simulink model "experiment_supervisor"  (R2023a)
settings: Solver=FixedStepDiscrete  StartTime=0.0  StopTime=inf  FixedStep=Ts  RelTol=1e-3
model workspace (MAT data in the model file):
  Ts = Simulink.Parameter
  Ts.Value = 0.01
  Ts.DataType = 'auto'
  Ts.DocUnits = 's'
  Ts.Complexity = 'real'
  Ts.Dimensions = [1 1]
  board_ID = Simulink.Parameter
  board_ID.Value = 1
  board_ID.DataType = 'auto'
  board_ID.Complexity = 'real'
  board_ID.Dimensions = [1 1]
undefined symbols (not defined in the file or in its folder): CAN_ANGLE_DEG2ICUB, CAN_VOLT_REF_GAIN, CAN_VOLT_REF_SHIFT, canChannel
libraries: canmsglib x12, canlib x4
settings Model: DataDictionary=EmbeddedBoardDD.sldd  Creator=upattacini  LastModifiedBy=mfussi
settings SolverCC: AlgebraicLoopSolver=TrustRegion  DecoupledContinuousIntegration=on  MinimalZcImpactIntegration=on
settings OptimizationCC: ReuseModelBlockBuffer=off  SimCompilerOptimization=on
settings DebuggingCC: UnconnectedInputMsg=warning  UnconnectedOutputMsg=warning  UnconnectedLineMsg=warning  ArithmeticOperatorsInVariantConditions=warning
settings HardwareCC: ProdBitPerLong=64  ProdHWDeviceType=Intel->x86-64 (Linux 64)
settings ModelReferenceCC: EnableRefExpFcnMdlSchedulingChecks=on
settings SFSimCC: SimUseLocalCustomCode=off  CustomCodeUndefinedFunction=UseInterfaceOnly
settings RTWCC: Description=Simulink Desktop Real-Time  SystemTargetFile=sldrt.tlc  TemplateMakefile=sldrt.tmf  RTWUseLocalCustomCode=off  RTWCompilerOptimization=on  DLArmComputeVersion=19.05
settings CodeAppCC: MaxIdLength=95
settings SimulinkDesktopRealTimeCC: TargetLibSuffix=_sldrt.a  TargetPreCompLibLocation=C:\Program Files\MATLAB\R2023a\toolbox\sldrt\lib\win64

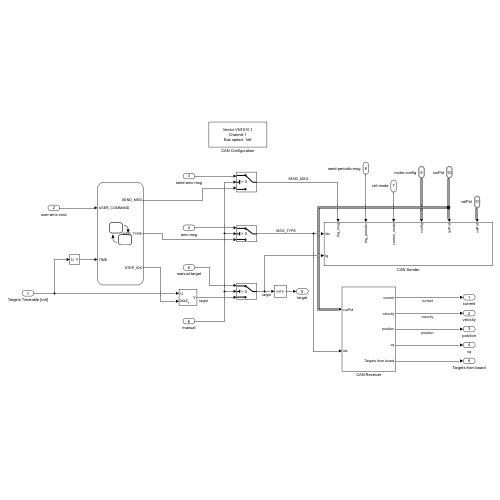
[thumbnail: Simulink's stored preview of the top-level diagram]
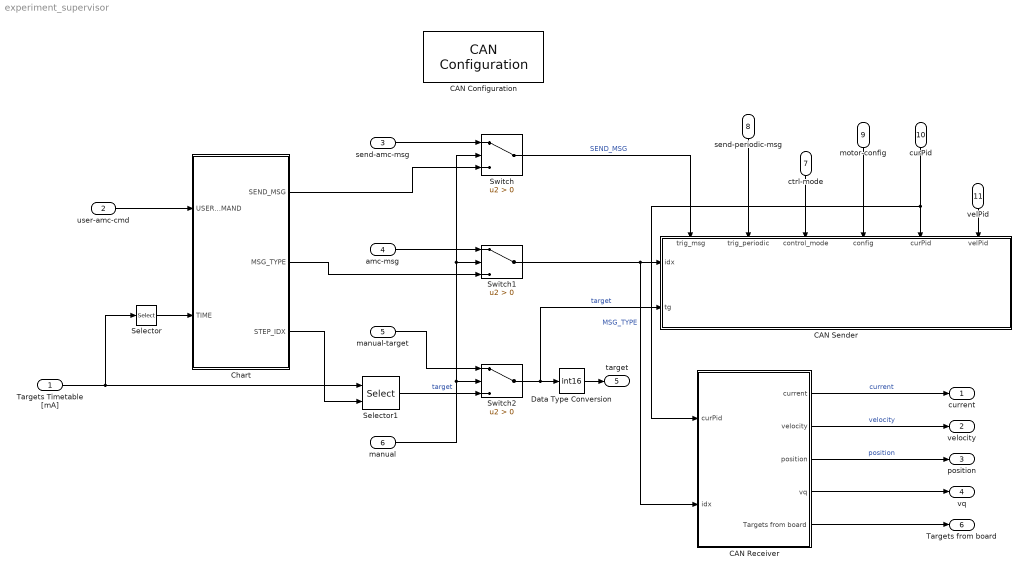
== system experiment_supervisor ==
  Targets Timetable [mA] : Inport  PortDimensions=[2, 8]
  user-amc-cmd : Inport  Port=2
  send-amc-msg : Inport  Port=3
  amc-msg : Inport  Port=4
  manual-target : Inport  Port=5
  manual : Inport  Port=6
  ctrl-mode : Inport  Port=7
  send-periodic-msg : Inport  Port=8
  motor-config : Inport  Port=9  OutDataTypeStr=Bus: MotorConfig
  curPid : Inport  Port=10  OutDataTypeStr=Bus: PIDConfig
  velPid : Inport  Port=11  OutDataTypeStr=Bus: PIDConfig
  CAN Configuration : canlib/CAN Configuration  BlockHandle=1472.0001  Device=Vector VN1610 1 (Channel 1)  DeviceMenu=Vector VN1610 1 (Channel 1)  ObjConstructor=canChannel('Vector', 'VN1610 1', 1)  BusSpeed=1e6  EnableBitParameters=off  SJW=1  TSEG1=4  TSEG2=3  NSamples=1  AckMode=Normal
  CAN Receiver : Subsystem
  CAN Sender : Subsystem
      settings: PortSchema="{\"entries\":[{\"content\":{\"sides\":[{\"content\":{\"connectorIds\":[\"In1\",\"In2\"]},\"type\":\"ConnectorPlacement.EquallySpacedRectSide\",\"uuid\":\"bdd6ce9e-9b65-4aba-9b48-f09f8c1326bb\"},{\"content\":{\"connectorIds\":[],\"side\":\"RIGHT\"},\"type\":\"ConnectorPlacement.EquallySpacedRectSide\",\"uuid\":\"141c9ef5-f742-47fc-b635-015c7474b58f\"},{\"content\":{\"connectorIds\":[\"In3\",\"In4\",\"In5\",\"In6\",\"In7\",\"In8\"],\"side\":\"TOP\"},\"type\":\"ConnectorPlacement.EquallySpacedRectSide\",\"uuid\":\"624889ac-74c5-4b05-9d21-0587daea952f\"}]},\"type\":\"ConnectorPlacement.EquallySpacedConnector\",\"uuid\":\"a748afda-e52d-41b4-a312-ee668058905d\"}],\"packageUris\":[\"http://schema.mathworks.com/mf0/Connector/R2020b\"],\"version\":\"1.0\"}"
  Chart : Stateflow chart  TreatAsAtomicUnit=on
      settings: PortSchema="{\"entries\":[{\"content\":{\"sides\":[{\"content\":{\"connectorIds\":[\"In1\",\"In2\"]},\"type\":\"ConnectorPlacement.EquallySpacedRectSide\",\"uuid\":\"3f3ecf7a-eca8-49e2-a594-4c8df01bcae2\"},{\"content\":{\"connectorIds\":[\"Out2\",\"Out1\",\"Out3\"],\"side\":\"RIGHT\"},\"type\":\"ConnectorPlacement.EquallySpacedRectSide\",\"uuid\":\"2e405059-6050-4daf-b42b-e1c8d6f3a572\"},{\"content\":{\"connectorIds\":[],\"side\":\"TOP\"},\"type\":\"ConnectorPlacement.EquallySpacedRectSide\",\"uuid\":\"8705f6e5-e301-4990-b24d-44270950b42f\"}]},\"type\":\"ConnectorPlacement.EquallySpacedConnector\",\"uuid\":\"46b9b7aa-14e0-48f8-b8fe-455c7835f2bb\"}],\"packageUris\":[\"http://schema.mathworks.com/mf0/Connector/R2020b\"],\"version\":\"1.0\"}"
  Data Type Conversion : DataTypeConversion  OutDataTypeStr=int16  SaturateOnIntegerOverflow=off  RndMeth=Floor
  Selector : Selector  NumberOfDimensions=2  InputPortWidth=2  IndexOptions=Index vector (dialog),Select all  Indices=1,2  OutputSizes=1,6
  Selector1 : Selector  NumberOfDimensions=2  InputPortWidth=2  IndexOptions=Index vector (dialog),Index vector (port)  Indices=2,2  OutputSizes=1,6
  Switch : Switch  Criteria=u2 > Threshold  SaturateOnIntegerOverflow=off  InputSameDT=off
  Switch1 : Switch  Criteria=u2 > Threshold  SaturateOnIntegerOverflow=off  InputSameDT=off
  Switch2 : Switch  Criteria=u2 > Threshold  SaturateOnIntegerOverflow=off  InputSameDT=off
  current : Outport
  velocity : Outport  Port=2
  position : Outport  Port=3
  vq : Outport  Port=4
  target : Outport  Port=5
  Targets from board : Outport  Port=6
  wires:
  Chart/1(MSG_TYPE) -> Switch1/3
  amc-msg/1 -> Switch1/1
  user-amc-cmd/1 -> Chart/1(USER_COMMAND)
  Chart/2(SEND_MSG) -> Switch/3
  send-amc-msg/1 -> Switch/1
  Switch/1 -> CAN Sender/3(trig_msg)  "SEND_MSG"
  Switch1/1 -> CAN Sender/1(idx), CAN Receiver/2(idx)  "MSG_TYPE"
  Chart/3(STEP_IDX) -> Selector1/2
  Selector/1 -> Chart/2(TIME)
  Switch2/1 -> Data Type Conversion/1, CAN Sender/2(tg)  "target"
  manual-target/1 -> Switch2/1
  Selector1/1 -> Switch2/3  "target"
  manual/1 -> Switch/2, Switch1/2, Switch2/2
  Targets Timetable [mA]/1 -> Selector/1, Selector1/1
  CAN Receiver/1(current) -> current/1  "current"
  CAN Receiver/2(velocity) -> velocity/1  "velocity"
  CAN Receiver/3(position) -> position/1  "position"
  CAN Receiver/4(vq) -> vq/1
  ctrl-mode/1 -> CAN Sender/5(control_mode)
  send-periodic-msg/1 -> CAN Sender/4(trig_periodic)
  Data Type Conversion/1 -> target/1
  CAN Receiver/5(Targets from board) -> Targets from board/1
  velPid/1 -> CAN Sender/8(velPid)
  curPid/1 -> CAN Sender/7(curPid), CAN Receiver/1(curPid)
  motor-config/1 -> CAN Sender/6(config)

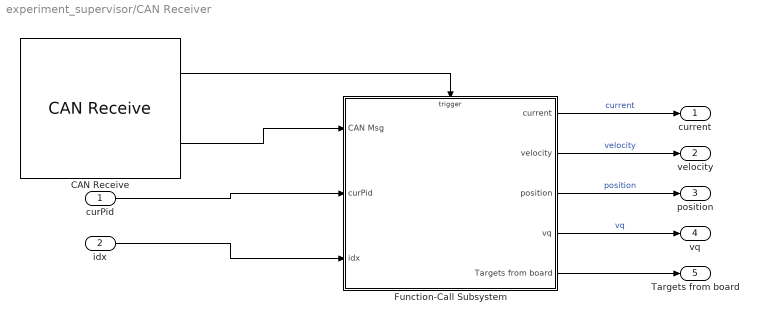
== system experiment_supervisor/CAN Receiver ==
  curPid : Inport  OutDataTypeStr=Bus: PIDConfig
  idx : Inport  Port=2
  CAN Receive : canlib/CAN Receive  BlockHandle=1483.0001  Device=Vector VN1610 1 (Channel 1)  DeviceMenu=Vector VN1610 1 (Channel 1)  ObjConstructor=canChannel('Vector', 'VN1610 1', 1)  EnableStandardIDsFilter=off  StdIDsCombo=Allow all  StandardIDs=0  EnableExtendedIDsFilter=off  ExtIDsCombo=Allow all  ExtendedIDs=0  SampleTime=Ts  MsgsPerTimestep=all  InternalFilterUpdateStatus=on  BusOutput=on
  Function-Call Subsystem : Subsystem  TreatAsAtomicUnit=on
  current : Outport
  velocity : Outport  Port=2
  position : Outport  Port=3
  vq : Outport  Port=4
  Targets from board : Outport  Port=5
  wires:
  CAN Receive/1 -> Function-Call Subsystem/Trigger
  CAN Receive/2 -> Function-Call Subsystem/1(CAN Msg)
  idx/1 -> Function-Call Subsystem/3(idx)
  Function-Call Subsystem/1(current) -> current/1  "current"
  Function-Call Subsystem/2(velocity) -> velocity/1  "velocity"
  Function-Call Subsystem/3(position) -> position/1  "position"
  Function-Call Subsystem/4(vq) -> vq/1  "vq"
  Function-Call Subsystem/5(Targets from board) -> Targets from board/1
  curPid/1 -> Function-Call Subsystem/2(curPid)

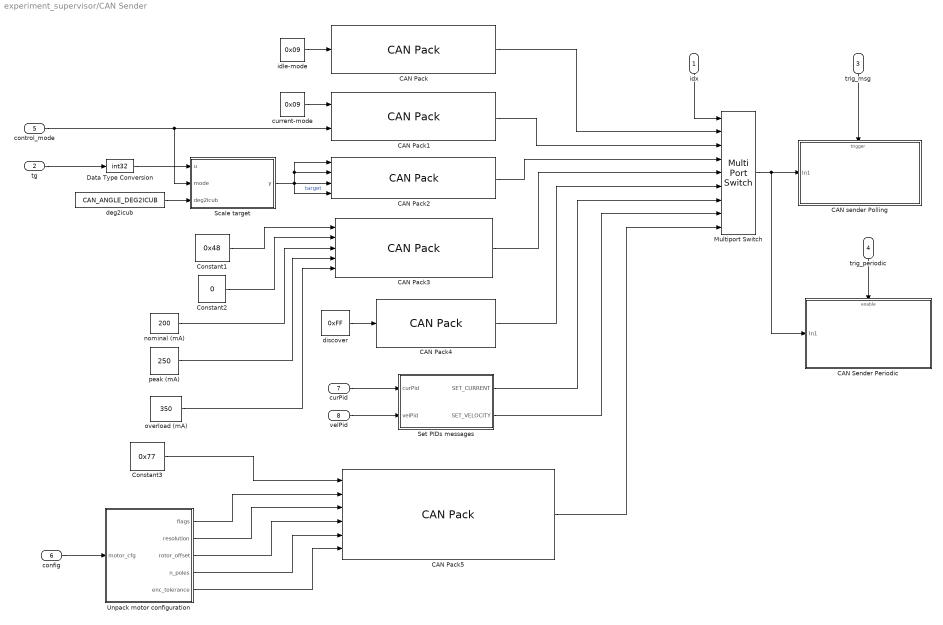
== system experiment_supervisor/CAN Sender ==
  idx : Inport
  tg : Inport  Port=2
  trig_msg : Inport  Port=3
  trig_periodic : Inport  Port=4
  control_mode : Inport  Port=5
  config : Inport  Port=6  OutDataTypeStr=Bus: MotorConfig
  curPid : Inport  Port=7
  velPid : Inport  Port=8
  CAN Pack : canmsglib/CAN Pack  MsgList=(none)  MsgName=CAN Idle  MsgIDType=Standard (11-bit identifier)  MsgIdentifier=board_ID  MsgLength=2  Remote=off  ApplyMinMax=off  BusOutput=on  SignalInfo={ 'Idle', '0', '16', 'LE', 'unsigned', 'Standard', '0', '1', '0', '-Inf', 'Inf' }
      settings: DataFormat=manually specified signals
  CAN Pack1 : canmsglib/CAN Pack  MsgList=(none)  MsgName=SET Control Mode  MsgIDType=Standard (11-bit identifier)  MsgIdentifier=board_ID  MsgLength=2  Remote=off  ApplyMinMax=off  BusOutput=on  SignalInfo={ 'CMD', '0', '8', 'LE', 'unsigned', 'Standard', '0', '1', '0', '-Inf', 'Inf'; 'CTRL', '8', '8', 'LE', 'signed', 'Standard', '0', '1', '0', '-Inf', 'Inf' }
      settings: DataFormat=manually specified signals
  CAN Pack2 : canmsglib/CAN Pack  MsgList=(none)  MsgName=CAN Target  MsgIDType=Standard (11-bit identifier)  MsgIdentifier=0x10F  MsgLength=8  Remote=off  ApplyMinMax=off  BusOutput=on  SignalInfo={ 'Target 1', '0', '16', 'LE', 'signed', 'Standard', '0', '1', '0', '-Inf', 'Inf'; 'Target 2', '16', '16', 'LE', 'signed', 'Standard', '0', '1', '0', '-Inf', 'Inf'; 'Target 3', '32', '16', 'LE', 'signed', 'Standard', '0', '1', '0', '-Inf', 'Inf'; 'Target 4', '48', '16', 'LE', 'signed', 'Standard', '0', '1', '0', '-Inf', 'Inf' }
      settings: DataFormat=manually specified signals
  CAN Pack3 : canmsglib/CAN Pack  MsgList=(none)  MsgName=CAN Limits  MsgIDType=Standard (11-bit identifier)  MsgIdentifier=board_ID  MsgLength=8  Remote=off  ApplyMinMax=off  BusOutput=on  SignalInfo={ 'CMD', '0', '8', 'LE', 'unsigned', 'Standard', '0', '1', '0', '-Inf', 'Inf'; 'X', '8', '8', 'LE', 'unsigned', 'Standard', '0', '1', '0', '-Inf', 'Inf'; 'NOMINAL', '16', '16', 'LE', 'unsigned', 'Standard', '0', '1', '0', '-Inf', 'Inf'; 'PEAK', '32', '16', 'LE', 'unsigned', 'Standard', '0', '1', '0', '-Inf', 'Inf'; 'OVERLOAD', '48', '16', 'LE', 'unsigned', 'Standard', '0', '1', '0', '-Inf', 'Inf' }
      settings: DataFormat=manually specified signals
  CAN Pack4 : canmsglib/CAN Pack  MsgList=(none)  MsgName=DISCOVER  MsgIDType=Standard (11-bit identifier)  MsgIdentifier=0x70F  MsgLength=1  Remote=off  ApplyMinMax=off  BusOutput=on  SignalInfo={}
      settings: DataFormat=raw data
  CAN Pack5 : canmsglib/CAN Pack  MsgList=(none)  MsgName=Set_Motor_Config  MsgIDType=Standard (11-bit identifier)  MsgIdentifier=board_ID  MsgLength=8  Remote=off  ApplyMinMax=off  BusOutput=on  SignalInfo={ 'CMD', '0', '8', 'LE', 'unsigned', 'Standard', '0', '1', '0', '-Inf', 'Inf'; 'FLAGS', '8', '8', 'LE', 'unsigned', 'Standard', '0', '1', '0', '-Inf', 'Inf'; 'RES_ENCODER', '16', '16', 'LE', 'signed', 'Standard', '0', '1', '0', '-Inf', 'Inf'; 'OFFSET_ENCODER', '32', '16', 'LE', 'unsigned', 'Standard', '0', '1', '0', '-Inf', 'Inf'; 'N_POLES', '48', '8', 'LE', 'unsigned', 'Standard', '0', '1', '0', '-Inf', 'Inf'; 'ENCODER_TOLERANCE', '56', '8', 'LE', 'unsigned', 'Standard', '0', '1', '0', '-Inf', 'Inf' }
      settings: DataFormat=manually specified signals
  CAN Sender Periodic : Subsystem  TreatAsAtomicUnit=on
  CAN sender Polling : Subsystem
  Constant1 : Constant  Value=0x48  OutDataTypeStr=Inherit: Inherit via back propagation
  Constant2 : Constant  Value=0  OutDataTypeStr=Inherit: Inherit via back propagation
  Constant3 : Constant  Value=0x77  OutDataTypeStr=Inherit: Inherit via back propagation
  Data Type Conversion : DataTypeConversion  OutDataTypeStr=int32  SaturateOnIntegerOverflow=off  RndMeth=Floor
  Multiport Switch : MultiPortSwitch  Inputs=8  DiagnosticForDefault=Warning  SaturateOnIntegerOverflow=off  InputSameDT=off
  Scale target : MATLAB Function  TreatAsAtomicUnit=on
  Set PIDs messages : Subsystem
  Unpack motor configuration : MATLAB Function  TreatAsAtomicUnit=on
  current-mode : Constant  Value=0x09  OutDataTypeStr=Inherit: Inherit via back propagation
  deg2icub : Constant  Value=CAN_ANGLE_DEG2ICUB
  discover : Constant  Value=0xFF
  idle-mode : Constant  Value=0x09  OutDataTypeStr=Inherit: Inherit via back propagation
  nominal (mA) : Constant  Value=200  OutDataTypeStr=Inherit: Inherit via back propagation
  overload (mA) : Constant  Value=350  OutDataTypeStr=Inherit: Inherit via back propagation
  peak (mA) : Constant  Value=250  OutDataTypeStr=Inherit: Inherit via back propagation
  wires:
  CAN Pack/1 -> Multiport Switch/2
  CAN Pack1/1 -> Multiport Switch/3
  CAN Pack2/1 -> Multiport Switch/4
  idx/1 -> Multiport Switch/1
  idle-mode/1 -> CAN Pack/1
  current-mode/1 -> CAN Pack1/1
  Constant1/1 -> CAN Pack3/1
  CAN Pack3/1 -> Multiport Switch/5
  discover/1 -> CAN Pack4/1
  CAN Pack4/1 -> Multiport Switch/6
  trig_msg/1 -> CAN sender Polling/Trigger
  Constant2/1 -> CAN Pack3/2
  nominal (mA)/1 -> CAN Pack3/3
  peak (mA)/1 -> CAN Pack3/4
  overload (mA)/1 -> CAN Pack3/5
  trig_periodic/1 -> CAN Sender Periodic/Enable
  Scale target/1(y) -> CAN Pack2/4, CAN Pack2/1, CAN Pack2/2, CAN Pack2/3  "target"
  Multiport Switch/1 -> CAN Sender Periodic/1(In1), CAN sender Polling/1(In1)
  control_mode/1 -> CAN Pack1/2, Scale target/2(mode)
  tg/1 -> Data Type Conversion/1
  Data Type Conversion/1 -> Scale target/1(u)
  Constant3/1 -> CAN Pack5/1
  Set PIDs messages/2(SET_VELOCITY) -> Multiport Switch/8
  Set PIDs messages/1(SET_CURRENT) -> Multiport Switch/7
  velPid/1 -> Set PIDs messages/2(velPid)
  CAN Pack5/1 -> Multiport Switch/9
  config/1 -> Unpack motor configuration/1(motor_cfg)
  curPid/1 -> Set PIDs messages/1(curPid)
  Unpack motor configuration/1(flags) -> CAN Pack5/2
  Unpack motor configuration/2(resolution) -> CAN Pack5/3
  Unpack motor configuration/3(rotor_offset) -> CAN Pack5/4
  Unpack motor configuration/4(n_poles) -> CAN Pack5/5
  Unpack motor configuration/5(enc_tolerance) -> CAN Pack5/6
  deg2icub/1 -> Scale target/3(deg2icub)

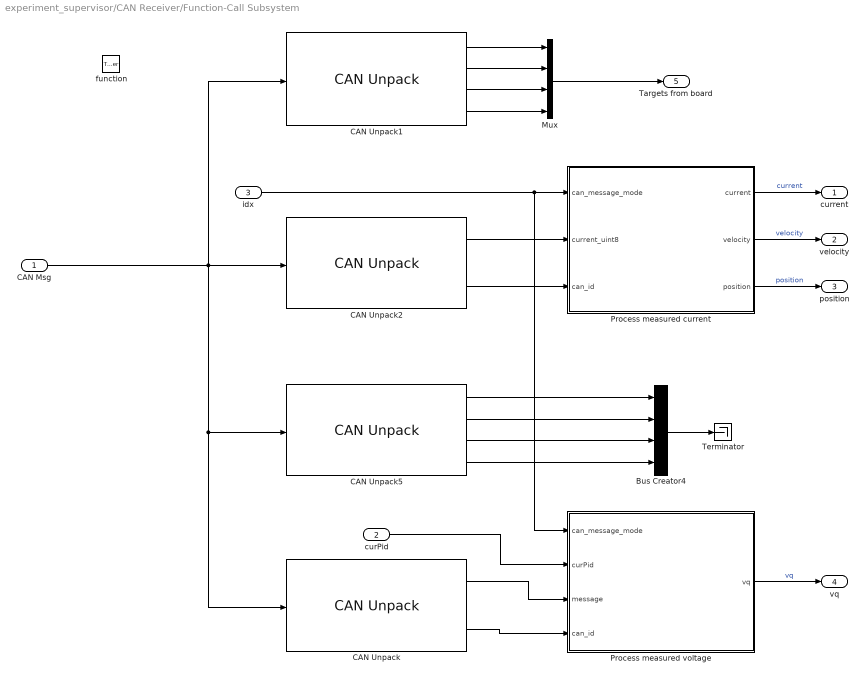
== system experiment_supervisor/CAN Receiver/Function-Call Subsystem ==
  CAN Msg : Inport
  curPid : Inport  Port=2  OutDataTypeStr=Bus: PIDConfig
  idx : Inport  Port=3
  function : TriggerPort  TriggerType=function-call  VariantControl=(inherit)
  Bus Creator4 : BusCreator  Inputs=4
  CAN Unpack : canmsglib/CAN Unpack  MsgList=(none)  MsgName=STATUS  MsgIDType=Standard (11-bit identifier)  MsgIdentifier=0x113  MsgLength=8  SignalInfo={}  IDPort=on  TimestampPort=off  ErrorPort=off  RemotePort=off  LengthPort=off  StatusPort=off  ApplyMinMax=off
      settings: DataFormat=raw data
  CAN Unpack1 : canmsglib/CAN Unpack  MsgList=(none)  MsgName=TARGETS  MsgIDType=Standard (11-bit identifier)  MsgIdentifier=0x10F  MsgLength=8  SignalInfo={ 'Target1', '0', '16', 'LE', 'signed', 'Standard', '0', '1', '0', '-Inf', 'Inf'; 'Target2', '16', '16', 'LE', 'signed', 'Standard', '0', '1', '0', '-Inf', 'Inf'; 'Target3', '32', '16', 'LE', 'signed', 'Standard', '0', '1', '0', '-Inf', 'Inf'; 'Target4', '48', '16', 'LE', 'signed', 'Standard', '0', '1', '0', '-Inf', 'Inf' }  IDPort=off  TimestampPort=off  ErrorPort=off  RemotePort=off  LengthPort=off  StatusPort=off  ApplyMinMax=off
  CAN Unpack2 : canmsglib/CAN Unpack  MsgList=(none)  MsgName=FOC  MsgIDType=Standard (11-bit identifier)  MsgIdentifier=0x110  MsgLength=8  SignalInfo={}  IDPort=on  TimestampPort=off  ErrorPort=off  RemotePort=off  LengthPort=off  StatusPort=off  ApplyMinMax=off
      settings: DataFormat=raw data
  CAN Unpack5 : canmsglib/CAN Unpack  MsgList=(none)  MsgName=DISCOVER  MsgIDType=Standard (11-bit identifier)  MsgIdentifier=0x710  MsgLength=5  SignalInfo={}  IDPort=on  TimestampPort=on  ErrorPort=off  RemotePort=off  LengthPort=on  StatusPort=off  ApplyMinMax=off
      settings: DataFormat=raw data
  Mux : Mux
  Process measured current : Subsystem
  Process measured voltage : Subsystem
  Terminator : Terminator
  current : Outport  Unit=mA
  velocity : Outport  Port=2
  position : Outport  Port=3
  vq : Outport  Port=4
  Targets from board : Outport  Port=5
  wires:
  CAN Msg/1 -> CAN Unpack1/1, CAN Unpack/1, CAN Unpack5/1, CAN Unpack2/1
  CAN Unpack2/1 -> Process measured current/2(current_uint8)
  CAN Unpack2/2 -> Process measured current/3(can_id)
  CAN Unpack5/4 -> Bus Creator4/4
  CAN Unpack5/3 -> Bus Creator4/3
  CAN Unpack5/2 -> Bus Creator4/2
  CAN Unpack5/1 -> Bus Creator4/1
  Bus Creator4/1 -> Terminator/1
  Process measured current/1(current) -> current/1  "current"
  idx/1 -> Process measured voltage/1(can_message_mode), Process measured current/1(can_message_mode)
  Process measured current/2(velocity) -> velocity/1  "velocity"
  Process measured current/3(position) -> position/1  "position"
  CAN Unpack/1 -> Process measured voltage/3(message)
  CAN Unpack/2 -> Process measured voltage/4(can_id)
  Process measured voltage/1(vq) -> vq/1  "vq"
  CAN Unpack1/1 -> Mux/1
  CAN Unpack1/2 -> Mux/2
  CAN Unpack1/3 -> Mux/3
  CAN Unpack1/4 -> Mux/4
  Mux/1 -> Targets from board/1
  curPid/1 -> Process measured voltage/2(curPid)

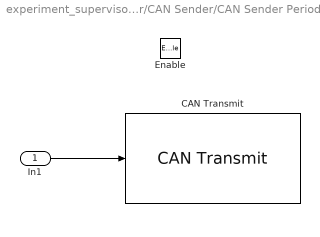
== system experiment_supervisor/CAN Sender/CAN Sender Periodic ==
  In1 : Inport
  Enable : EnablePort
  CAN Transmit : canlib/CAN Transmit  BlockHandle=1115.0001  Device=Vector VN1610 1 (Channel 1)  DeviceMenu=Vector VN1610 1 (Channel 1)  ObjConstructor=canChannel('Vector', 'VN1610 1', 1)  EnableEventTransmit=off  EnablePeriodicTransmit=on  MessagePeriod=Ts
  wires:
  In1/1 -> CAN Transmit/1

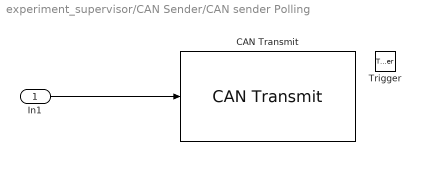
== system experiment_supervisor/CAN Sender/CAN sender Polling ==
  In1 : Inport
  Trigger : TriggerPort  VariantControl=(inherit)  PortDimensions=1
  CAN Transmit : canlib/CAN Transmit  BlockHandle=1123.0001  Device=Vector VN1610 1 (Channel 1)  DeviceMenu=Vector VN1610 1 (Channel 1)  ObjConstructor=canChannel('Vector', 'VN1610 1', 1)  EnableEventTransmit=off  EnablePeriodicTransmit=off  MessagePeriod=1.000
  wires:
  In1/1 -> CAN Transmit/1

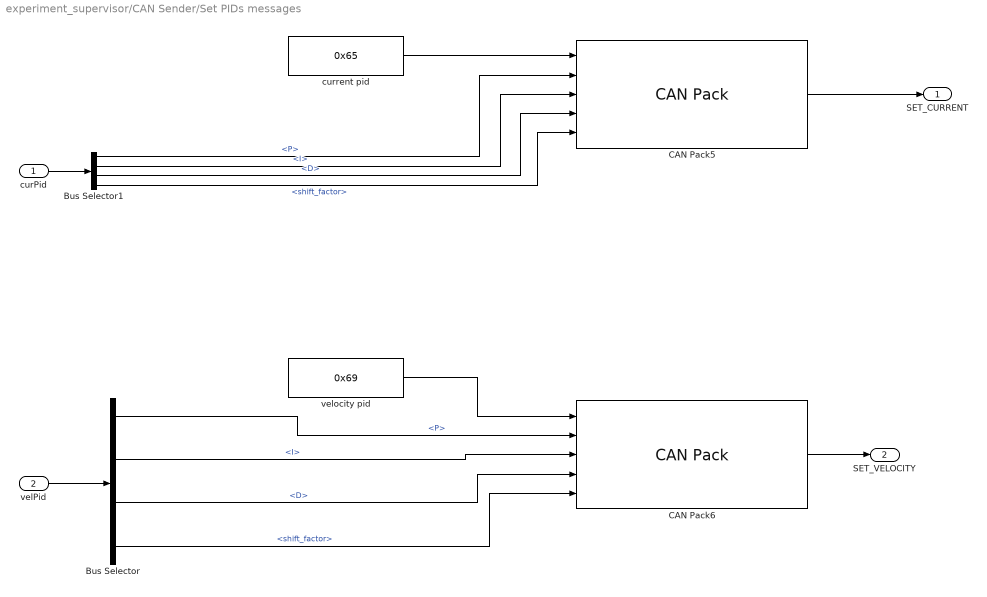
== system experiment_supervisor/CAN Sender/Set PIDs messages ==
  curPid : Inport
  velPid : Inport  Port=2  OutDataTypeStr=Bus: PIDConfig
  Bus Selector : BusSelector  OutputSignals=P,I,D,shift_factor
  Bus Selector1 : BusSelector  OutputSignals=P,I,D,shift_factor
  CAN Pack5 : canmsglib/CAN Pack  MsgList=(none)  MsgName=SET_CURRENT_PID  MsgIDType=Standard (11-bit identifier)  MsgIdentifier=board_ID  MsgLength=8  Remote=off  ApplyMinMax=off  BusOutput=on  SignalInfo={ 'CMD', '0', '8', 'LE', 'unsigned', 'Standard', '0', '1', '0', '-Inf', 'Inf'; 'Kp', '8', '16', 'LE', 'signed', 'Standard', '0', '1', '0', '-Inf', 'Inf'; 'Ki', '24', '16', 'LE', 'signed', 'Standard', '0', '1', '0', '-Inf', 'Inf'; 'Kd', '40', '16', 'LE', 'signed', 'Standard', '0', '1', '0', '-Inf', 'Inf'; 'shift', '56', '8', 'LE', 'unsigned', 'Standard', '0', '1', '0', '-Inf', 'Inf' }
      settings: DataFormat=manually specified signals
  CAN Pack6 : canmsglib/CAN Pack  MsgList=(none)  MsgName=SET_VELOCITY_PID  MsgIDType=Standard (11-bit identifier)  MsgIdentifier=board_ID  MsgLength=8  Remote=off  ApplyMinMax=off  BusOutput=on  SignalInfo={ 'CMD', '0', '8', 'LE', 'unsigned', 'Standard', '0', '1', '0', '-Inf', 'Inf'; 'Kp', '8', '16', 'LE', 'signed', 'Standard', '0', '1', '0', '-Inf', 'Inf'; 'Ki', '24', '16', 'LE', 'signed', 'Standard', '0', '1', '0', '-Inf', 'Inf'; 'Kd', '40', '16', 'LE', 'signed', 'Standard', '0', '1', '0', '-Inf', 'Inf'; 'shift', '56', '8', 'LE', 'unsigned', 'Standard', '0', '1', '0', '-Inf', 'Inf' }
      settings: DataFormat=manually specified signals
  current pid : Constant  Value=0x65  OutDataTypeStr=int16
  velocity pid : Constant  Value=0x69  OutDataTypeStr=int16
  SET_CURRENT : Outport
  SET_VELOCITY : Outport  Port=2
  wires:
  Bus Selector/4 -> CAN Pack6/5  "<shift_factor>"
  Bus Selector/1 -> CAN Pack6/2  "<P>"
  Bus Selector1/4 -> CAN Pack5/5  "<shift_factor>"
  Bus Selector1/1 -> CAN Pack5/2  "<P>"
  Bus Selector/3 -> CAN Pack6/4  "<D>"
  Bus Selector/2 -> CAN Pack6/3  "<I>"
  Bus Selector1/2 -> CAN Pack5/3  "<I>"
  current pid/1 -> CAN Pack5/1
  velocity pid/1 -> CAN Pack6/1
  CAN Pack5/1 -> SET_CURRENT/1
  CAN Pack6/1 -> SET_VELOCITY/1
  velPid/1 -> Bus Selector/1
  curPid/1 -> Bus Selector1/1
  Bus Selector1/3 -> CAN Pack5/4  "<D>"

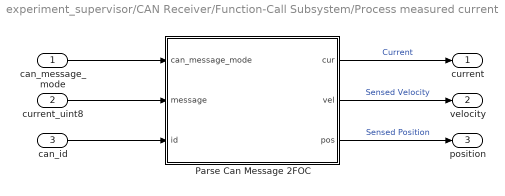
== system experiment_supervisor/CAN Receiver/Function-Call Subsystem/Process measured current ==
  can_message_mode : Inport
  current_uint8 : Inport  Port=2
  can_id : Inport  Port=3
  Parse Can Message 2FOC : MATLAB Function  TreatAsAtomicUnit=on
  current : Outport
  velocity : Outport  Port=2
  position : Outport  Port=3
  wires:
  Parse Can Message 2FOC/1(cur) -> current/1  "Current"
  current_uint8/1 -> Parse Can Message 2FOC/2(message)
  Parse Can Message 2FOC/2(vel) -> velocity/1  "Sensed Velocity"
  Parse Can Message 2FOC/3(pos) -> position/1  "Sensed Position"
  can_id/1 -> Parse Can Message 2FOC/3(id)
  can_message_mode/1 -> Parse Can Message 2FOC/1(can_message_mode)

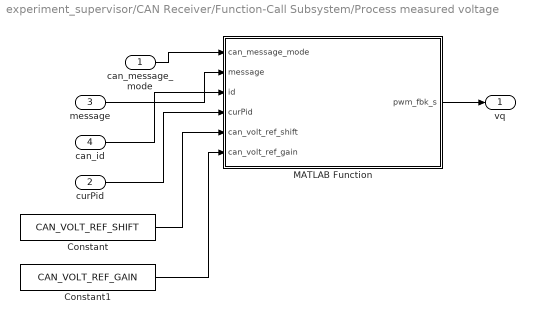
== system experiment_supervisor/CAN Receiver/Function-Call Subsystem/Process measured voltage ==
  can_message_mode : Inport
  curPid : Inport  Port=2  OutDataTypeStr=Bus: PIDConfig
  message : Inport  Port=3
  can_id : Inport  Port=4
  Constant : Constant  Value=CAN_VOLT_REF_SHIFT
  Constant1 : Constant  Value=CAN_VOLT_REF_GAIN
  MATLAB Function : MATLAB Function  TreatAsAtomicUnit=on
  vq : Outport  OutDataTypeStr=single  PortDimensions=1
  wires:
  can_message_mode/1 -> MATLAB Function/1(can_message_mode)
  MATLAB Function/1(pwm_fbk_s) -> vq/1
  message/1 -> MATLAB Function/2(message)
  can_id/1 -> MATLAB Function/3(id)
  curPid/1 -> MATLAB Function/4(curPid)
  Constant/1 -> MATLAB Function/5(can_volt_ref_shift)
  Constant1/1 -> MATLAB Function/6(can_volt_ref_gain)

== matlab function experiment_supervisor/CAN Sender/Unpack motor configuration ==
  data: flags output; resolution output; rotor_offset output; n_poles output; motor_cfg input; enc_tolerance output
function [flags, resolution,rotor_offset, n_poles, enc_tolerance] = unpack_cfg(motor_cfg)

    flags = uint8(motor_cfg.has_quadrature_encoder); 
    flags = bitor(flags, bitshift(uint8(motor_cfg.has_hall_sens), 1));
    resolution = motor_cfg.rotor_encoder_resolution;
    rotor_offset = motor_cfg.rotor_index_offset;
    n_poles = motor_cfg.pole_pairs * 2;
    enc_tolerance = motor_cfg.encoder_tolerance;

end

== matlab function experiment_supervisor/CAN Sender/Scale target ==
  data: u input; y output; mode input; deg2icub input
function y = fcn(u, mode, deg2icub)

switch mode
    case 0x0A % velocity control mode
        y = u / (deg2icub * 1000); 
    case 0x50 % voltage control mode
        y = bitshift(u * 10, 5);
    otherwise
        y =  u;
end

== stateflow chart experiment_supervisor/Chart ==
  state RESET_IDLE
    entry:
    SEND_MSG=1;
    STEP_IDX=1;
    on after(1, sec):
    SEND_MSG=0;
  state WAIT_LIMITS
    entry:
    SEND_MSG=1;
    on after(1, sec):
    SEND_MSG=0;
  state IDLE
    entry:
    SEND_MSG=1;
    STEP_IDX=1;
    on after(1 , sec):
    SEND_MSG=0;
  state STARTED
    entry:
    SEND_MSG=1;
    on after(1 , sec):
    SEND_MSG=0;
  state WAIT_CTRL_MODE
    entry:
    SEND_MSG=1;
    on after(1,sec):
    SEND_MSG=0;
  (default) -> RESET_IDLE
  STARTED -> RESET_IDLE [order 4] : [USER_COMMAND == 2]
      | {MSG_TYPE = 1;}
  RESET_IDLE -> WAIT_LIMITS [order 1] : [USER_COMMAND == 1]
      | {MSG_TYPE = 4;}
  IDLE -> RESET_IDLE [order 2] : [USER_COMMAND == 2]
      | {MSG_TYPE=1;}
  WAIT_LIMITS -> RESET_IDLE [order 2] : [USER_COMMAND == 2]
      | {MSG_TYPE = 1;}
  RESET_IDLE -> RESET_IDLE [order 2] : [USER_COMMAND == 2]
      | {MSG_TYPE=1;}
  WAIT_CTRL_MODE -> RESET_IDLE [order 2] : [USER_COMMAND == 2]
      | {MSG_TYPE = 1;}
  IDLE -> IDLE [order 3] : [USER_COMMAND == 0 ]
      | {MSG_TYPE=1;}
  WAIT_LIMITS -> WAIT_CTRL_MODE [order 1] : after(2, sec){MSG_TYPE = 2;}
  STARTED -> IDLE [order 2] : [USER_COMMAND == 0 ]
      | {MSG_TYPE=1;}
  IDLE -> WAIT_CTRL_MODE [order 1] : [USER_COMMAND == 1]
      | {MSG_TYPE = 2;}
  WAIT_CTRL_MODE -> STARTED [order 1] : after(2, sec){MSG_TYPE=3;
      | STEP_IDX=1;}
  STARTED -> STARTED [order 1] : after(TIME(STEP_IDX), sec)[STEP_IDX <length(TIME)]
      | {STEP_IDX = STEP_IDX + 1;}
  STARTED -> STARTED [order 3] : [USER_COMMAND == 1]{MSG_TYPE = 3;}
  data: MSG_TYPE output uint8 =uint8(1); USER_COMMAND input; SEND_MSG output uint8 =uint8(0); TIME input; STEP_IDX output uint32 =uint32(1)

== matlab function experiment_supervisor/CAN Receiver/Function-Call Subsystem/Process measured current/Parse Can Message 2FOC ==
  data: can_message_mode input; message input; cur output; vel output; pos output; id input; CAN_ANGLE_ICUB2DEG parameter
function [cur, vel, pos] = parse_can_message_2foc(can_message_mode, message, id, CAN_ANGLE_ICUB2DEG)

foc_message_id = 0x120;

persistent prev_cur
persistent prev_pos
persistent prev_vel

% initialization
if isempty(prev_cur)
    prev_cur = int16(0);
end
if isempty(prev_pos)
    prev_pos = single(0);
end
if isempty(prev_vel)
    prev_vel = single(0);
end

% reset value when (re)start
if(can_message_mode == 1 || can_message_mode == 4)
    cur = int16(0);
    vel = single(0);
    
    prev_cur = cur;
    prev_vel = vel;
    pos = prev_pos;
    
elseif (id == foc_message_id)
    cur = typecast(uint8([message(1), message(2)]), 'int16');
    vel = single(typecast(uint8([message(3), message(4)]), 'int16'));
    pos = single(typecast(uint8([message(5), message(6), message(7), message(8)]), 'int32'));
    
    % units conversion:
    % - pos from icubdeg to deg
    % - vel from icubdeg/ms to deg/s
    pos = pos * CAN_ANGLE_ICUB2DEG ;
    vel = vel * CAN_ANGLE_ICUB2DEG * 1000;
    
    prev_cur = cur;
    prev_pos = pos;
    prev_vel = vel;
    
else
    cur = prev_cur;
    vel = prev_vel;
    pos = prev_pos;
end


end

== matlab function experiment_supervisor/CAN Receiver/Function-Call Subsystem/Process measured voltage/MATLAB Function ==
  data: can_message_mode input; pwm_fbk_s output; message input; id input; curPid input; can_volt_ref_shift input; can_volt_ref_gain input
function pwm_fbk_s  = parse_can_message_status(can_message_mode, message, id, curPid, can_volt_ref_shift, can_volt_ref_gain)

status_message_id = 0x123;

persistent prev_pwm_fbk

% initialization
if isempty(prev_pwm_fbk)
    prev_pwm_fbk = int16(0);
end

% reset value when (re)start
if(can_message_mode == 1 || can_message_mode == 4)
    pwm_fbk = int16(0);

% parse the message
elseif (id == status_message_id)

    pwm_fbk = typecast(uint8([message(3), message(4)]), 'int16');
    prev_pwm_fbk = pwm_fbk;

else
    pwm_fbk = prev_pwm_fbk;
end
    pwm_fbk_s = single(bitshift(pwm_fbk, curPid.shift_factor - can_volt_ref_shift)) /can_volt_ref_gain; % 5 = CAN_VOLT_REF_SHIFT
end
